simulink model "NUgus"  (R2018a)
settings: Solver=VariableStepAuto  StartTime=0.0  StopTime=inf  RelTol=1e-2
values from neighbouring files (symbols this model uses):
  CM740_acc_bias = 4 * 9.80743    (= 39.22972)    [CM740_init.m]
  CM740_acc_gain = 512 / CM740_acc_centre    [CM740_init.m]
  CM740_gyro_bias = 1600 / 360 * 2 * pi    (= 27.9252680319)    [CM740_init.m]
  CM740_gyro_gain = 512 / CM740_gyro_centre    [CM740_init.m]
  g = 9.8107    [init.m]
  head = [-0.05482228998067195, -0.00010888238321339966, 0.0011712900228573724, 0.41900000000000004]    [comtest.m]
  Kw = 0.9    [init.m]
  model = NUgusKinematics()    [KinematicsTest.m]    (also in Support_Region.m; init.m = NUgusKinematics)
  period = 1.0    (= 1)    [init.m]
  s = mean(abs(present_speed.data))    [RunServoTest.m]
  sample_time = 1/90    (= 0.0111111111111)    [init.m]
  step_height = 0.1    [init.m]
  torso = [0.0050079703254699804, 0.008880921777563762, 0.1021503146237477, 2.5390000000000006]    [comtest.m]
  z0 = 0.45    [init.m]
undefined symbols (not defined in the file or in its folder): sigbuilder_block, X, Y, Z
libraries: sm_lib x206, nesl_utility x82, Contact_Forces_Lib x10
(part 6 of 7)

== system NUgus/NUgus/right_upper_arm ==
  Inertia : sm_lib/Body Elements/Inertia  InertiaType=Custom  Mass=model.mass.arm_upper(4)  MassUnits=kg  CenterOfMass=[0, 0, 0]  CenterOfMassUnits=m  MomentsOfInertia=[model.inertia.upper_arm(1,1), model.inertia.upper_arm(2,2), model.inertia.upper_arm(3,3)]  MomentsOfInertiaUnits=kg*m^2  ProductsOfInertia=-[model.inertia.upper_arm(2,3), model.inertia.upper_arm(3,1), model.inertia.upper_arm(1,2)]  ProductsOfInertiaUnits=kg*m^2  GraphicType=Marker  MarkerShape=Inertia  MarkerSize=20  GraphicVisPropType=SimpleVisualProperties  GraphicDiffuseColor=[0.8 0.8 0.8]  GraphicSpecularColor=[0.5 0.5 0.5 1.0]  GraphicAmbientColor=[0.15 0.15 0.15 1.0]  GraphicEmissiveColor=[0.0 0.0 0.0 1.0]  GraphicShininess=75  GraphicOpacity=inertia_opacity
  InertiaOriginTransform : sm_lib/Frames and Transforms/Rigid Transform  TranslationMethod=Cartesian  TranslationStandardOffset=0  TranslationLengthUnit=m  TranslationStandardAxis=+Z  TranslationCartesianOffset=[0.006723 -0.090631 0.000549]  TranslationROffset=0  TranslationROffsetUnits=m  TranslationZOffset=0  TranslationZOffsetUnits=m  TranslationThetaOffset=0  TranslationThetaOffsetUnits=deg  RotationMethod=RotationSequence  RotationAngleUnits=deg  RotationStandardAxis=+Z  RotationAngle=0.0  RotationArbitraryAxis=[0 0 1]  FollAlignAxisA=+X  BaseAlignAxisA=+Y  FollAlignAxisB=+Y  BaseAlignAxisB=+Z  RotationSequenceAxes=BaseAxes  RotationSequence=XYZ  RotationSequenceAngles=[0, 0, 0]  RotationSequenceAnglesUnits=rad  RotationMatrix=[1 0 0; 0 1 0; 0 0 1]
  ReferenceFrame : sm_lib/Frames and Transforms/Reference Frame
  right_elbow_pitch_AxisTransform : sm_lib/Frames and Transforms/Rigid Transform  TranslationMethod=Cartesian  TranslationStandardOffset=0  TranslationLengthUnit=m  TranslationStandardAxis=+Z  TranslationCartesianOffset=[0, 0, 0]  TranslationROffset=0  TranslationROffsetUnits=m  TranslationZOffset=0  TranslationZOffsetUnits=m  TranslationThetaOffset=0  TranslationThetaOffsetUnits=deg  RotationMethod=ArbitraryAxis  RotationAngleUnits=rad  RotationStandardAxis=+Z  RotationAngle=1.570796326794897  RotationArbitraryAxis=[-0, 1, 0]  FollAlignAxisA=+X  BaseAlignAxisA=+Y  FollAlignAxisB=+Y  BaseAlignAxisB=+Z  RotationSequenceAxes=FollowerAxes  RotationSequence=XYX  RotationSequenceAngles=[0 0 0]  RotationSequenceAnglesUnits=deg  RotationMatrix=[1 0 0; 0 1 0; 0 0 1]
  right_elbow_pitch_OriginTransform : sm_lib/Frames and Transforms/Rigid Transform  TranslationMethod=Cartesian  TranslationStandardOffset=0  TranslationLengthUnit=m  TranslationStandardAxis=+Z  TranslationCartesianOffset=[0.01, -0.19, 0.04]  TranslationROffset=0  TranslationROffsetUnits=m  TranslationZOffset=0  TranslationZOffsetUnits=m  TranslationThetaOffset=0  TranslationThetaOffsetUnits=deg  RotationMethod=RotationSequence  RotationAngleUnits=deg  RotationStandardAxis=+Z  RotationAngle=0.0  RotationArbitraryAxis=[0 0 1]  FollAlignAxisA=+X  BaseAlignAxisA=+Y  FollAlignAxisB=+Y  BaseAlignAxisB=+Z  RotationSequenceAxes=BaseAxes  RotationSequence=XYZ  RotationSequenceAngles=[0, 0, 0]  RotationSequenceAnglesUnits=rad  RotationMatrix=[1 0 0; 0 1 0; 0 0 1]
  right_shoulder_roll_AxisInvTransform : sm_lib/Frames and Transforms/Rigid Transform  TranslationMethod=Cartesian  TranslationStandardOffset=0  TranslationLengthUnit=m  TranslationStandardAxis=+Z  TranslationCartesianOffset=[0, 0, 0]  TranslationROffset=0  TranslationROffsetUnits=m  TranslationZOffset=0  TranslationZOffsetUnits=m  TranslationThetaOffset=0  TranslationThetaOffsetUnits=deg  RotationMethod=ArbitraryAxis  RotationAngleUnits=rad  RotationStandardAxis=+Z  RotationAngle=0  RotationArbitraryAxis=[1, 0, 0]  FollAlignAxisA=+X  BaseAlignAxisA=+Y  FollAlignAxisB=+Y  BaseAlignAxisB=+Z  RotationSequenceAxes=FollowerAxes  RotationSequence=XYX  RotationSequenceAngles=[0 0 0]  RotationSequenceAnglesUnits=deg  RotationMatrix=[1 0 0; 0 1 0; 0 0 1]
  right_upper_arm_visual : sm_lib/Body Elements/Solid  InertiaType=Custom  Mass=0  MassUnits=kg  CenterOfMass=[0, 0, 0]  CenterOfMassUnits=m  MomentsOfInertia=[0, 0, 0]  MomentsOfInertiaUnits=kg*m^2  ProductsOfInertia=[0, 0, 0]  ProductsOfInertiaUnits=kg*m^2  DensityBased=on  Density=1000  DensityUnits=kg/m^3  DoExposeReferenceFrame=on  SerializedFrames=<Frames/>  GraphicType=FromGeometry  MarkerShape=Sphere  MarkerSize=10  GraphicVisPropType=SimpleVisualProperties  GraphicDiffuseColor=[0.5, 0.5, 0.5]  GraphicSpecularColor=[0.5 0.5 0.5 1.0]  GraphicAmbientColor=[0.15 0.15 0.15 1.0]  GraphicEmissiveColor=[0.0 0.0 0.0 1.0]  GraphicShininess=75  GraphicOpacity=1  GeometryShape=FromFile  RectangleSize=[1 1]  RectangleSizeUnits=m  BrickDimensions=[1 1 1]  BrickDimensionUnits=m  CylinderRadius=1  CylinderRadiusUnits=m  CylinderLength=1  CylinderLengthUnits=m  SphereRadius=1  SphereRadiusUnits=m  EllipsoidRadii=[1 1 1]  EllipsoidRadiiUnits=m  ExtrusionCrossSection=[1 1; -1 1; -1 -1; 1 -1]  ExtrusionCrossSectionUnits=m  ExtrusionLength=1  ExtrusionLengthUnits=m  PolygonNumSides=3  PolygonOuterRadius=1  PolygonOuterRadiusUnits=m  ExtGeomFileType=STL  ExtGeomFileName=mesh/right_upper_arm.stl  ExtGeomFileUnits=m  RevolutionCrossSection=[1 1; 1 -1; 2 -1; 2 1]  RevolutionCrossSectionUnits=m  RevolutionExtent=Full  RevolutionAngle=180  RevolutionAngleUnits=deg
  right_upper_arm_visualOriginTransform : sm_lib/Frames and Transforms/Rigid Transform  TranslationMethod=Cartesian  TranslationStandardOffset=0  TranslationLengthUnit=m  TranslationStandardAxis=+Z  TranslationCartesianOffset=[0, 0, 0]  TranslationROffset=0  TranslationROffsetUnits=m  TranslationZOffset=0  TranslationZOffsetUnits=m  TranslationThetaOffset=0  TranslationThetaOffsetUnits=deg  RotationMethod=RotationSequence  RotationAngleUnits=deg  RotationStandardAxis=+Z  RotationAngle=0.0  RotationArbitraryAxis=[0 0 1]  FollAlignAxisA=+X  BaseAlignAxisA=+Y  FollAlignAxisB=+Y  BaseAlignAxisB=+Z  RotationSequenceAxes=BaseAxes  RotationSequence=XYZ  RotationSequenceAngles=[0, 0, 0]  RotationSequenceAnglesUnits=rad  RotationMatrix=[1 0 0; 0 1 0; 0 0 1]
  F : PMIOPort  Side=Left
  F1 : PMIOPort  Port=2  Side=Right
  connections:
  Inertia/RConn1 -- InertiaOriginTransform/RConn1
  ReferenceFrame/RConn1 -- InertiaOriginTransform/LConn1 -- right_elbow_pitch_OriginTransform/LConn1 -- right_shoulder_roll_AxisInvTransform/LConn1 -- right_upper_arm_visualOriginTransform/LConn1
  right_elbow_pitch_AxisTransform/RConn1 -- F1/RConn1
  right_elbow_pitch_AxisTransform/LConn1 -- right_elbow_pitch_OriginTransform/RConn1
  right_shoulder_roll_AxisInvTransform/RConn1 -- F/RConn1
  right_upper_arm_visual/RConn1 -- right_upper_arm_visualOriginTransform/RConn1

== system NUgus/NUgus/right_upper_leg ==
  Inertia : sm_lib/Body Elements/Inertia  InertiaType=Custom  Mass=model.mass.leg_upper(4)  MassUnits=kg  CenterOfMass=[0, 0, 0]  CenterOfMassUnits=m  MomentsOfInertia=[model.inertia.upper_leg(1,1), model.inertia.upper_leg(2,2), model.inertia.upper_leg(3,3)]  MomentsOfInertiaUnits=kg*m^2  ProductsOfInertia=-[model.inertia.upper_leg(2,3), model.inertia.upper_leg(3,1), model.inertia.upper_leg(1,2)]  ProductsOfInertiaUnits=kg*m^2  GraphicType=Marker  MarkerShape=Inertia  MarkerSize=20  GraphicVisPropType=SimpleVisualProperties  GraphicDiffuseColor=[0.8 0.8 0.8]  GraphicSpecularColor=[0.5 0.5 0.5 1.0]  GraphicAmbientColor=[0.15 0.15 0.15 1.0]  GraphicEmissiveColor=[0.0 0.0 0.0 1.0]  GraphicShininess=75  GraphicOpacity=inertia_opacity
  InertiaOriginTransform : sm_lib/Frames and Transforms/Rigid Transform  TranslationMethod=Cartesian  TranslationStandardOffset=0  TranslationLengthUnit=m  TranslationStandardAxis=+Z  TranslationCartesianOffset=[0.000592 -0.005444 -0.102193]  TranslationROffset=0  TranslationROffsetUnits=m  TranslationZOffset=0  TranslationZOffsetUnits=m  TranslationThetaOffset=0  TranslationThetaOffsetUnits=deg  RotationMethod=RotationSequence  RotationAngleUnits=deg  RotationStandardAxis=+Z  RotationAngle=0.0  RotationArbitraryAxis=[0 0 1]  FollAlignAxisA=+X  BaseAlignAxisA=+Y  FollAlignAxisB=+Y  BaseAlignAxisB=+Z  RotationSequenceAxes=BaseAxes  RotationSequence=XYZ  RotationSequenceAngles=[0, 0, 0]  RotationSequenceAnglesUnits=rad  RotationMatrix=[1 0 0; 0 1 0; 0 0 1]
  ReferenceFrame : sm_lib/Frames and Transforms/Reference Frame
  right_hip_pitch_AxisInvTransform : sm_lib/Frames and Transforms/Rigid Transform  TranslationMethod=Cartesian  TranslationStandardOffset=0  TranslationLengthUnit=m  TranslationStandardAxis=+Z  TranslationCartesianOffset=[0, 0, 0]  TranslationROffset=0  TranslationROffsetUnits=m  TranslationZOffset=0  TranslationZOffsetUnits=m  TranslationThetaOffset=0  TranslationThetaOffsetUnits=deg  RotationMethod=ArbitraryAxis  RotationAngleUnits=rad  RotationStandardAxis=+Z  RotationAngle=1.570796326794897  RotationArbitraryAxis=[-0, 1, 0]  FollAlignAxisA=+X  BaseAlignAxisA=+Y  FollAlignAxisB=+Y  BaseAlignAxisB=+Z  RotationSequenceAxes=FollowerAxes  RotationSequence=XYX  RotationSequenceAngles=[0 0 0]  RotationSequenceAnglesUnits=deg  RotationMatrix=[1 0 0; 0 1 0; 0 0 1]
  right_knee_pitch_AxisTransform : sm_lib/Frames and Transforms/Rigid Transform  TranslationMethod=Cartesian  TranslationStandardOffset=0  TranslationLengthUnit=m  TranslationStandardAxis=+Z  TranslationCartesianOffset=[0, 0, 0]  TranslationROffset=0  TranslationROffsetUnits=m  TranslationZOffset=0  TranslationZOffsetUnits=m  TranslationThetaOffset=0  TranslationThetaOffsetUnits=deg  RotationMethod=ArbitraryAxis  RotationAngleUnits=rad  RotationStandardAxis=+Z  RotationAngle=1.570796326794897  RotationArbitraryAxis=[-0, 1, 0]  FollAlignAxisA=+X  BaseAlignAxisA=+Y  FollAlignAxisB=+Y  BaseAlignAxisB=+Z  RotationSequenceAxes=FollowerAxes  RotationSequence=XYX  RotationSequenceAngles=[0 0 0]  RotationSequenceAnglesUnits=deg  RotationMatrix=[1 0 0; 0 1 0; 0 0 1]
  right_knee_pitch_OriginTransform : sm_lib/Frames and Transforms/Rigid Transform  TranslationMethod=Cartesian  TranslationStandardOffset=0  TranslationLengthUnit=m  TranslationStandardAxis=+Z  TranslationCartesianOffset=[0, 0, -0.18976]  TranslationROffset=0  TranslationROffsetUnits=m  TranslationZOffset=0  TranslationZOffsetUnits=m  TranslationThetaOffset=0  TranslationThetaOffsetUnits=deg  RotationMethod=RotationSequence  RotationAngleUnits=deg  RotationStandardAxis=+Z  RotationAngle=0.0  RotationArbitraryAxis=[0 0 1]  FollAlignAxisA=+X  BaseAlignAxisA=+Y  FollAlignAxisB=+Y  BaseAlignAxisB=+Z  RotationSequenceAxes=BaseAxes  RotationSequence=XYZ  RotationSequenceAngles=[0.05, 0, 0]  RotationSequenceAnglesUnits=rad  RotationMatrix=[1 0 0; 0 1 0; 0 0 1]
  right_upper_leg_visual : sm_lib/Body Elements/Solid  InertiaType=Custom  Mass=0  MassUnits=kg  CenterOfMass=[0, 0, 0]  CenterOfMassUnits=m  MomentsOfInertia=[0, 0, 0]  MomentsOfInertiaUnits=kg*m^2  ProductsOfInertia=[0, 0, 0]  ProductsOfInertiaUnits=kg*m^2  DensityBased=on  Density=1000  DensityUnits=kg/m^3  DoExposeReferenceFrame=on  SerializedFrames=<Frames/>  GraphicType=FromGeometry  MarkerShape=Sphere  MarkerSize=10  GraphicVisPropType=SimpleVisualProperties  GraphicDiffuseColor=[0.5, 0.5, 0.5]  GraphicSpecularColor=[0.5 0.5 0.5 1.0]  GraphicAmbientColor=[0.15 0.15 0.15 1.0]  GraphicEmissiveColor=[0.0 0.0 0.0 1.0]  GraphicShininess=75  GraphicOpacity=1  GeometryShape=FromFile  RectangleSize=[1 1]  RectangleSizeUnits=m  BrickDimensions=[1 1 1]  BrickDimensionUnits=m  CylinderRadius=1  CylinderRadiusUnits=m  CylinderLength=1  CylinderLengthUnits=m  SphereRadius=1  SphereRadiusUnits=m  EllipsoidRadii=[1 1 1]  EllipsoidRadiiUnits=m  ExtrusionCrossSection=[1 1; -1 1; -1 -1; 1 -1]  ExtrusionCrossSectionUnits=m  ExtrusionLength=1  ExtrusionLengthUnits=m  PolygonNumSides=3  PolygonOuterRadius=1  PolygonOuterRadiusUnits=m  ExtGeomFileType=STL  ExtGeomFileName=mesh/right_upper_leg.stl  ExtGeomFileUnits=m  RevolutionCrossSection=[1 1; 1 -1; 2 -1; 2 1]  RevolutionCrossSectionUnits=m  RevolutionExtent=Full  RevolutionAngle=180  RevolutionAngleUnits=deg
  right_upper_leg_visualOriginTransform : sm_lib/Frames and Transforms/Rigid Transform  TranslationMethod=Cartesian  TranslationStandardOffset=0  TranslationLengthUnit=m  TranslationStandardAxis=+Z  TranslationCartesianOffset=[0, 0, 0]  TranslationROffset=0  TranslationROffsetUnits=m  TranslationZOffset=0  TranslationZOffsetUnits=m  TranslationThetaOffset=0  TranslationThetaOffsetUnits=deg  RotationMethod=RotationSequence  RotationAngleUnits=deg  RotationStandardAxis=+Z  RotationAngle=0.0  RotationArbitraryAxis=[0 0 1]  FollAlignAxisA=+X  BaseAlignAxisA=+Y  FollAlignAxisB=+Y  BaseAlignAxisB=+Z  RotationSequenceAxes=BaseAxes  RotationSequence=XYZ  RotationSequenceAngles=[0, 0, 0]  RotationSequenceAnglesUnits=rad  RotationMatrix=[1 0 0; 0 1 0; 0 0 1]
  F : PMIOPort  Side=Left
  F1 : PMIOPort  Port=2  Side=Right
  connections:
  Inertia/RConn1 -- InertiaOriginTransform/RConn1
  ReferenceFrame/RConn1 -- InertiaOriginTransform/LConn1 -- right_hip_pitch_AxisInvTransform/LConn1 -- right_knee_pitch_OriginTransform/LConn1 -- right_upper_leg_visualOriginTransform/LConn1
  right_hip_pitch_AxisInvTransform/RConn1 -- F/RConn1
  right_knee_pitch_AxisTransform/RConn1 -- F1/RConn1
  right_knee_pitch_AxisTransform/LConn1 -- right_knee_pitch_OriginTransform/RConn1
  right_upper_leg_visual/RConn1 -- right_upper_leg_visualOriginTransform/RConn1

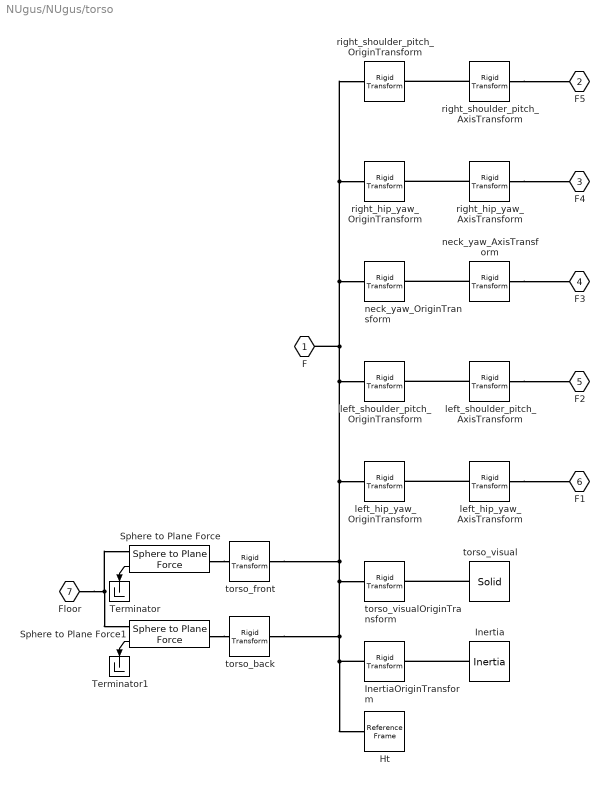
== system NUgus/NUgus/torso ==
  Ht : sm_lib/Frames and Transforms/Reference Frame
  Inertia : sm_lib/Body Elements/Inertia  InertiaType=Custom  Mass=model.mass.torso(4)  MassUnits=kg  CenterOfMass=[0, 0, 0]  CenterOfMassUnits=m  MomentsOfInertia=[model.inertia.torso(1,1), model.inertia.torso(2,2), model.inertia.torso(3,3)]  MomentsOfInertiaUnits=kg*m^2  ProductsOfInertia=-[model.inertia.torso(2,3), model.inertia.torso(3,1), model.inertia.torso(1,2)]  ProductsOfInertiaUnits=kg*m^2  GraphicType=Marker  MarkerShape=Inertia  MarkerSize=20  GraphicVisPropType=SimpleVisualProperties  GraphicDiffuseColor=[0.8 0.8 0.8]  GraphicSpecularColor=[0.5 0.5 0.5 1.0]  GraphicAmbientColor=[0.15 0.15 0.15 1.0]  GraphicEmissiveColor=[0.0 0.0 0.0 1.0]  GraphicShininess=75  GraphicOpacity=inertia_opacity
  InertiaOriginTransform : sm_lib/Frames and Transforms/Rigid Transform  TranslationMethod=Cartesian  TranslationStandardOffset=0  TranslationLengthUnit=m  TranslationStandardAxis=+Z  TranslationCartesianOffset=[-0.000000 0.000339 0.112557]  TranslationROffset=0  TranslationROffsetUnits=m  TranslationZOffset=0  TranslationZOffsetUnits=m  TranslationThetaOffset=0  TranslationThetaOffsetUnits=deg  RotationMethod=RotationSequence  RotationAngleUnits=deg  RotationStandardAxis=+Z  RotationAngle=0.0  RotationArbitraryAxis=[0 0 1]  FollAlignAxisA=+X  BaseAlignAxisA=+Y  FollAlignAxisB=+Y  BaseAlignAxisB=+Z  RotationSequenceAxes=BaseAxes  RotationSequence=XYZ  RotationSequenceAngles=[0, 0, 0]  RotationSequenceAnglesUnits=rad  RotationMatrix=[1 0 0; 0 1 0; 0 0 1]
  Sphere to Plane Force : Contact_Forces_Lib/3D/Sphere to Plane Force  sphere_rad=floor.stud_radius  plane_lenx=floor.length  plane_leny=floor.width  plane_depth=floor.depth/2  force_law=Linear  k_contact=floor.contact_stiffness  b_contact=floor.contact_damping  pen_full_damp_F=1e-4  pen_exponent=1  custom_param_1=1  custom_param_2=1  friction_law=Stick-Slip Continuous  mu_kinetic=floor.kinetic_friction  mu_static=floor.static_friction  v_thr=floor.vel_gain  vis_on=off  vis_opc_en=0  vis_len_plaBz=0.005  vis_clr=[0.9 0.2 0.2]  vis_opc=0.7
  Sphere to Plane Force1 : Contact_Forces_Lib/3D/Sphere to Plane Force  sphere_rad=floor.stud_radius  plane_lenx=floor.length  plane_leny=floor.width  plane_depth=floor.depth/2  force_law=Linear  k_contact=floor.contact_stiffness  b_contact=floor.contact_damping  pen_full_damp_F=1e-4  pen_exponent=1  custom_param_1=1  custom_param_2=1  friction_law=Stick-Slip Continuous  mu_kinetic=floor.kinetic_friction  mu_static=floor.static_friction  v_thr=floor.vel_gain  vis_on=off  vis_opc_en=0  vis_len_plaBz=0.005  vis_clr=[0.9 0.2 0.2]  vis_opc=0.7
  Terminator : Terminator
  Terminator1 : Terminator
  left_hip_yaw_AxisTransform : sm_lib/Frames and Transforms/Rigid Transform  TranslationMethod=Cartesian  TranslationStandardOffset=0  TranslationLengthUnit=m  TranslationStandardAxis=+Z  TranslationCartesianOffset=[0, 0, 0]  TranslationROffset=0  TranslationROffsetUnits=m  TranslationZOffset=0  TranslationZOffsetUnits=m  TranslationThetaOffset=0  TranslationThetaOffsetUnits=deg  RotationMethod=ArbitraryAxis  RotationAngleUnits=rad  RotationStandardAxis=+Z  RotationAngle=0  RotationArbitraryAxis=[1, 0, 0]  FollAlignAxisA=+X  BaseAlignAxisA=+Y  FollAlignAxisB=+Y  BaseAlignAxisB=+Z  RotationSequenceAxes=FollowerAxes  RotationSequence=XYX  RotationSequenceAngles=[0 0 0]  RotationSequenceAnglesUnits=deg  RotationMatrix=[1 0 0; 0 1 0; 0 0 1]
  left_hip_yaw_OriginTransform : sm_lib/Frames and Transforms/Rigid Transform  TranslationMethod=Cartesian  TranslationStandardOffset=0  TranslationLengthUnit=m  TranslationStandardAxis=+Z  TranslationCartesianOffset=[0, 0.055, 0]  TranslationROffset=0  TranslationROffsetUnits=m  TranslationZOffset=0  TranslationZOffsetUnits=m  TranslationThetaOffset=0  TranslationThetaOffsetUnits=deg  RotationMethod=RotationSequence  RotationAngleUnits=deg  RotationStandardAxis=+Z  RotationAngle=0.0  RotationArbitraryAxis=[0 0 1]  FollAlignAxisA=+X  BaseAlignAxisA=+Y  FollAlignAxisB=+Y  BaseAlignAxisB=+Z  RotationSequenceAxes=BaseAxes  RotationSequence=XYZ  RotationSequenceAngles=[0, 0, 1.57079]  RotationSequenceAnglesUnits=rad  RotationMatrix=[1 0 0; 0 1 0; 0 0 1]
  left_shoulder_pitch_AxisTransform : sm_lib/Frames and Transforms/Rigid Transform  TranslationMethod=Cartesian  TranslationStandardOffset=0  TranslationLengthUnit=m  TranslationStandardAxis=+Z  TranslationCartesianOffset=[0, 0, 0]  TranslationROffset=0  TranslationROffsetUnits=m  TranslationZOffset=0  TranslationZOffsetUnits=m  TranslationThetaOffset=0  TranslationThetaOffsetUnits=deg  RotationMethod=ArbitraryAxis  RotationAngleUnits=rad  RotationStandardAxis=+Z  RotationAngle=1.570796326794897  RotationArbitraryAxis=[-0, 1, 0]  FollAlignAxisA=+X  BaseAlignAxisA=+Y  FollAlignAxisB=+Y  BaseAlignAxisB=+Z  RotationSequenceAxes=FollowerAxes  RotationSequence=XYX  RotationSequenceAngles=[0 0 0]  RotationSequenceAnglesUnits=deg  RotationMatrix=[1 0 0; 0 1 0; 0 0 1]
  left_shoulder_pitch_OriginTransform : sm_lib/Frames and Transforms/Rigid Transform  TranslationMethod=Cartesian  TranslationStandardOffset=0  TranslationLengthUnit=m  TranslationStandardAxis=+Z  TranslationCartesianOffset=[0.005, 0.115, 0.18]  TranslationROffset=0  TranslationROffsetUnits=m  TranslationZOffset=0  TranslationZOffsetUnits=m  TranslationThetaOffset=0  TranslationThetaOffsetUnits=deg  RotationMethod=RotationSequence  RotationAngleUnits=deg  RotationStandardAxis=+Z  RotationAngle=0.0  RotationArbitraryAxis=[0 0 1]  FollAlignAxisA=+X  BaseAlignAxisA=+Y  FollAlignAxisB=+Y  BaseAlignAxisB=+Z  RotationSequenceAxes=BaseAxes  RotationSequence=XYZ  RotationSequenceAngles=[-1.57079, 0, 1.57079]  RotationSequenceAnglesUnits=rad  RotationMatrix=[1 0 0; 0 1 0; 0 0 1]
  neck_yaw_AxisTransform : sm_lib/Frames and Transforms/Rigid Transform  TranslationMethod=Cartesian  TranslationStandardOffset=0  TranslationLengthUnit=m  TranslationStandardAxis=+Z  TranslationCartesianOffset=[0, 0, 0]  TranslationROffset=0  TranslationROffsetUnits=m  TranslationZOffset=0  TranslationZOffsetUnits=m  TranslationThetaOffset=0  TranslationThetaOffsetUnits=deg  RotationMethod=ArbitraryAxis  RotationAngleUnits=rad  RotationStandardAxis=+Z  RotationAngle=0  RotationArbitraryAxis=[1, 0, 0]  FollAlignAxisA=+X  BaseAlignAxisA=+Y  FollAlignAxisB=+Y  BaseAlignAxisB=+Z  RotationSequenceAxes=FollowerAxes  RotationSequence=XYX  RotationSequenceAngles=[0 0 0]  RotationSequenceAnglesUnits=deg  RotationMatrix=[1 0 0; 0 1 0; 0 0 1]
  neck_yaw_OriginTransform : sm_lib/Frames and Transforms/Rigid Transform  TranslationMethod=Cartesian  TranslationStandardOffset=0  TranslationLengthUnit=m  TranslationStandardAxis=+Z  TranslationCartesianOffset=[0, 0, 0.26]  TranslationROffset=0  TranslationROffsetUnits=m  TranslationZOffset=0  TranslationZOffsetUnits=m  TranslationThetaOffset=0  TranslationThetaOffsetUnits=deg  RotationMethod=RotationSequence  RotationAngleUnits=deg  RotationStandardAxis=+Z  RotationAngle=0.0  RotationArbitraryAxis=[0 0 1]  FollAlignAxisA=+X  BaseAlignAxisA=+Y  FollAlignAxisB=+Y  BaseAlignAxisB=+Z  RotationSequenceAxes=BaseAxes  RotationSequence=XYZ  RotationSequenceAngles=[0, 0, 1.57079]  RotationSequenceAnglesUnits=rad  RotationMatrix=[1 0 0; 0 1 0; 0 0 1]
  right_hip_yaw_AxisTransform : sm_lib/Frames and Transforms/Rigid Transform  TranslationMethod=Cartesian  TranslationStandardOffset=0  TranslationLengthUnit=m  TranslationStandardAxis=+Z  TranslationCartesianOffset=[0, 0, 0]  TranslationROffset=0  TranslationROffsetUnits=m  TranslationZOffset=0  TranslationZOffsetUnits=m  TranslationThetaOffset=0  TranslationThetaOffsetUnits=deg  RotationMethod=ArbitraryAxis  RotationAngleUnits=rad  RotationStandardAxis=+Z  RotationAngle=0  RotationArbitraryAxis=[1, 0, 0]  FollAlignAxisA=+X  BaseAlignAxisA=+Y  FollAlignAxisB=+Y  BaseAlignAxisB=+Z  RotationSequenceAxes=FollowerAxes  RotationSequence=XYX  RotationSequenceAngles=[0 0 0]  RotationSequenceAnglesUnits=deg  RotationMatrix=[1 0 0; 0 1 0; 0 0 1]
  right_hip_yaw_OriginTransform : sm_lib/Frames and Transforms/Rigid Transform  TranslationMethod=Cartesian  TranslationStandardOffset=0  TranslationLengthUnit=m  TranslationStandardAxis=+Z  TranslationCartesianOffset=[0, -0.055, 0]  TranslationROffset=0  TranslationROffsetUnits=m  TranslationZOffset=0  TranslationZOffsetUnits=m  TranslationThetaOffset=0  TranslationThetaOffsetUnits=deg  RotationMethod=RotationSequence  RotationAngleUnits=deg  RotationStandardAxis=+Z  RotationAngle=0.0  RotationArbitraryAxis=[0 0 1]  FollAlignAxisA=+X  BaseAlignAxisA=+Y  FollAlignAxisB=+Y  BaseAlignAxisB=+Z  RotationSequenceAxes=BaseAxes  RotationSequence=XYZ  RotationSequenceAngles=[0, 0, 1.57079]  RotationSequenceAnglesUnits=rad  RotationMatrix=[1 0 0; 0 1 0; 0 0 1]
  right_shoulder_pitch_AxisTransform : sm_lib/Frames and Transforms/Rigid Transform  TranslationMethod=Cartesian  TranslationStandardOffset=0  TranslationLengthUnit=m  TranslationStandardAxis=+Z  TranslationCartesianOffset=[0, 0, 0]  TranslationROffset=0  TranslationROffsetUnits=m  TranslationZOffset=0  TranslationZOffsetUnits=m  TranslationThetaOffset=0  TranslationThetaOffsetUnits=deg  RotationMethod=ArbitraryAxis  RotationAngleUnits=rad  RotationStandardAxis=+Z  RotationAngle=1.570796326794897  RotationArbitraryAxis=[-0, 1, 0]  FollAlignAxisA=+X  BaseAlignAxisA=+Y  FollAlignAxisB=+Y  BaseAlignAxisB=+Z  RotationSequenceAxes=FollowerAxes  RotationSequence=XYX  RotationSequenceAngles=[0 0 0]  RotationSequenceAnglesUnits=deg  RotationMatrix=[1 0 0; 0 1 0; 0 0 1]
  right_shoulder_pitch_OriginTransform : sm_lib/Frames and Transforms/Rigid Transform  TranslationMethod=Cartesian  TranslationStandardOffset=0  TranslationLengthUnit=m  TranslationStandardAxis=+Z  TranslationCartesianOffset=[0.005, -0.115, 0.18]  TranslationROffset=0  TranslationROffsetUnits=m  TranslationZOffset=0  TranslationZOffsetUnits=m  TranslationThetaOffset=0  TranslationThetaOffsetUnits=deg  RotationMethod=RotationSequence  RotationAngleUnits=deg  RotationStandardAxis=+Z  RotationAngle=0.0  RotationArbitraryAxis=[0 0 1]  FollAlignAxisA=+X  BaseAlignAxisA=+Y  FollAlignAxisB=+Y  BaseAlignAxisB=+Z  RotationSequenceAxes=BaseAxes  RotationSequence=XYZ  RotationSequenceAngles=[-1.57079, 0, 1.57079]  RotationSequenceAnglesUnits=rad  RotationMatrix=[1 0 0; 0 1 0; 0 0 1]
  torso_back : sm_lib/Frames and Transforms/Rigid Transform  TranslationMethod=Cartesian  TranslationStandardOffset=0  TranslationLengthUnit=m  TranslationStandardAxis=+Z  TranslationCartesianOffset=[-0.069 0 0.15]  TranslationROffset=0  TranslationROffsetUnits=m  TranslationZOffset=0  TranslationZOffsetUnits=m  TranslationThetaOffset=0  TranslationThetaOffsetUnits=deg  RotationMethod=None  RotationAngleUnits=deg  RotationStandardAxis=+Z  RotationAngle=0.0  RotationArbitraryAxis=[0 0 1]  FollAlignAxisA=+X  BaseAlignAxisA=+Y  FollAlignAxisB=+Y  BaseAlignAxisB=+Z  RotationSequenceAxes=FollowerAxes  RotationSequence=XYX  RotationSequenceAngles=[0 0 0]  RotationSequenceAnglesUnits=deg  RotationMatrix=[1 0 0; 0 1 0; 0 0 1]
  torso_front : sm_lib/Frames and Transforms/Rigid Transform  TranslationMethod=Cartesian  TranslationStandardOffset=0  TranslationLengthUnit=m  TranslationStandardAxis=+Z  TranslationCartesianOffset=[0.067 0 0.15]  TranslationROffset=0  TranslationROffsetUnits=m  TranslationZOffset=0  TranslationZOffsetUnits=m  TranslationThetaOffset=0  TranslationThetaOffsetUnits=deg  RotationMethod=None  RotationAngleUnits=deg  RotationStandardAxis=+Z  RotationAngle=0.0  RotationArbitraryAxis=[0 0 1]  FollAlignAxisA=+X  BaseAlignAxisA=+Y  FollAlignAxisB=+Y  BaseAlignAxisB=+Z  RotationSequenceAxes=FollowerAxes  RotationSequence=XYX  RotationSequenceAngles=[0 0 0]  RotationSequenceAnglesUnits=deg  RotationMatrix=[1 0 0; 0 1 0; 0 0 1]
  torso_visual : sm_lib/Body Elements/Solid  InertiaType=Custom  Mass=0  MassUnits=kg  CenterOfMass=[0, 0, 0]  CenterOfMassUnits=m  MomentsOfInertia=[0, 0, 0]  MomentsOfInertiaUnits=kg*m^2  ProductsOfInertia=[0, 0, 0]  ProductsOfInertiaUnits=kg*m^2  DensityBased=on  Density=1000  DensityUnits=kg/m^3  DoExposeReferenceFrame=on  SerializedFrames=<Frames/>  GraphicType=FromGeometry  MarkerShape=Sphere  MarkerSize=10  GraphicVisPropType=SimpleVisualProperties  GraphicDiffuseColor=[0.5, 0.5, 0.5]  GraphicSpecularColor=[0.5 0.5 0.5 1.0]  GraphicAmbientColor=[0.15 0.15 0.15 1.0]  GraphicEmissiveColor=[0.0 0.0 0.0 1.0]  GraphicShininess=75  GraphicOpacity=1  GeometryShape=FromFile  RectangleSize=[1 1]  RectangleSizeUnits=m  BrickDimensions=[1 1 1]  BrickDimensionUnits=m  CylinderRadius=1  CylinderRadiusUnits=m  CylinderLength=1  CylinderLengthUnits=m  SphereRadius=1  SphereRadiusUnits=m  EllipsoidRadii=[1 1 1]  EllipsoidRadiiUnits=m  ExtrusionCrossSection=[1 1; -1 1; -1 -1; 1 -1]  ExtrusionCrossSectionUnits=m  ExtrusionLength=1  ExtrusionLengthUnits=m  PolygonNumSides=3  PolygonOuterRadius=1  PolygonOuterRadiusUnits=m  ExtGeomFileType=STL  ExtGeomFileName=mesh/torso.stl  ExtGeomFileUnits=m  RevolutionCrossSection=[1 1; 1 -1; 2 -1; 2 1]  RevolutionCrossSectionUnits=m  RevolutionExtent=Full  RevolutionAngle=180  RevolutionAngleUnits=deg
  torso_visualOriginTransform : sm_lib/Frames and Transforms/Rigid Transform  TranslationMethod=Cartesian  TranslationStandardOffset=0  TranslationLengthUnit=m  TranslationStandardAxis=+Z  TranslationCartesianOffset=[0, 0, 0]  TranslationROffset=0  TranslationROffsetUnits=m  TranslationZOffset=0  TranslationZOffsetUnits=m  TranslationThetaOffset=0  TranslationThetaOffsetUnits=deg  RotationMethod=RotationSequence  RotationAngleUnits=deg  RotationStandardAxis=+Z  RotationAngle=0.0  RotationArbitraryAxis=[0 0 1]  FollAlignAxisA=+X  BaseAlignAxisA=+Y  FollAlignAxisB=+Y  BaseAlignAxisB=+Z  RotationSequenceAxes=BaseAxes  RotationSequence=XYZ  RotationSequenceAngles=[0, 0, 1.57079]  RotationSequenceAnglesUnits=rad  RotationMatrix=[1 0 0; 0 1 0; 0 0 1]
  F : PMIOPort  Side=Left
  F5 : PMIOPort  Port=2  Side=Right
  F4 : PMIOPort  Port=3  Side=Right
  F3 : PMIOPort  Port=4  Side=Right
  F2 : PMIOPort  Port=5  Side=Right
  F1 : PMIOPort  Port=6  Side=Right
  Floor : PMIOPort  Port=7  Side=Left
  wires:
  Sphere to Plane Force/1 -> Terminator/1
  Sphere to Plane Force1/1 -> Terminator1/1
  connections:
  Inertia/RConn1 -- InertiaOriginTransform/RConn1
  InertiaOriginTransform/LConn1 -- Ht/RConn1 -- torso_back/LConn1 -- torso_front/LConn1 -- F/RConn1 -- right_hip_yaw_OriginTransform/LConn1 -- right_shoulder_pitch_OriginTransform/LConn1 -- neck_yaw_OriginTransform/LConn1 -- left_shoulder_pitch_OriginTransform/LConn1 -- left_hip_yaw_OriginTransform/LConn1 -- torso_visualOriginTransform/LConn1
  left_hip_yaw_AxisTransform/RConn1 -- F1/RConn1
  left_hip_yaw_AxisTransform/LConn1 -- left_hip_yaw_OriginTransform/RConn1
  left_shoulder_pitch_AxisTransform/RConn1 -- F2/RConn1
  left_shoulder_pitch_AxisTransform/LConn1 -- left_shoulder_pitch_OriginTransform/RConn1
  neck_yaw_AxisTransform/RConn1 -- F3/RConn1
  neck_yaw_AxisTransform/LConn1 -- neck_yaw_OriginTransform/RConn1
  right_hip_yaw_AxisTransform/RConn1 -- F4/RConn1
  right_hip_yaw_AxisTransform/LConn1 -- right_hip_yaw_OriginTransform/RConn1
  right_shoulder_pitch_AxisTransform/RConn1 -- F5/RConn1
  right_shoulder_pitch_AxisTransform/LConn1 -- right_shoulder_pitch_OriginTransform/RConn1
  torso_visual/RConn1 -- torso_visualOriginTransform/RConn1
  Sphere to Plane Force/LConn1 -- torso_front/RConn1
  Sphere to Plane Force1/LConn1 -- torso_back/RConn1
  Floor/RConn1 -- Sphere to Plane Force1/RConn1 -- Sphere to Plane Force/RConn1

== system NUgus/Control/Capture Step/Subsystem3 ==
  v3 : Inport
  Constant4 : Constant
  Demux5 : Demux  Outputs=3
  Mux2 : Mux
  v4 : Outport
  wires:
  Mux2/1 -> v4/1
  v3/1 -> Demux5/1
  Demux5/2 -> Mux2/2
  Demux5/3 -> Mux2/3
  Demux5/1 -> Mux2/1
  Constant4/1 -> Mux2/4

== system NUgus/Control/Capture Step/Subsystem4 ==
  v4 : Inport
  Demux5 : Demux
  Mux2 : Mux  Inputs=3
  Terminator : Terminator
  v3 : Outport
  wires:
  Mux2/1 -> v3/1
  v4/1 -> Demux5/1
  Demux5/2 -> Mux2/2
  Demux5/3 -> Mux2/3
  Demux5/1 -> Mux2/1
  Demux5/4 -> Terminator/1

== system NUgus/Control/ZMP/to real ==
  discrete : Inport
  Add : Sum  Inputs=+-
  Constant : Constant  Value=512
  Gain : Gain  Gain=(4 * 9.80657) / 512
  continuous : Outport
  wires:
  discrete/1 -> Add/1
  Add/1 -> Gain/1
  Gain/1 -> continuous/1
  Constant/1 -> Add/2

== system NUgus/Control/world to torso/Subsystem3 ==
  v3 : Inport
  Constant4 : Constant
  Demux5 : Demux  Outputs=3
  Mux2 : Mux
  v4 : Outport
  wires:
  Mux2/1 -> v4/1
  v3/1 -> Demux5/1
  Demux5/2 -> Mux2/2
  Demux5/3 -> Mux2/3
  Demux5/1 -> Mux2/1
  Constant4/1 -> Mux2/4

== system NUgus/Control/world to torso/Subsystem4 ==
  v4 : Inport
  Demux5 : Demux
  Mux2 : Mux  Inputs=3
  Terminator : Terminator
  v3 : Outport
  wires:
  Mux2/1 -> v3/1
  v4/1 -> Demux5/1
  Demux5/2 -> Mux2/2
  Demux5/3 -> Mux2/3
  Demux5/1 -> Mux2/1
  Demux5/4 -> Terminator/1

== system NUgus/Control/world to torso1/Subsystem3 ==
  v3 : Inport
  Constant4 : Constant
  Demux5 : Demux  Outputs=3
  Mux2 : Mux
  v4 : Outport
  wires:
  Mux2/1 -> v4/1
  v3/1 -> Demux5/1
  Demux5/2 -> Mux2/2
  Demux5/3 -> Mux2/3
  Demux5/1 -> Mux2/1
  Constant4/1 -> Mux2/4

== system NUgus/Control/world to torso1/Subsystem4 ==
  v4 : Inport
  Demux5 : Demux
  Mux2 : Mux  Inputs=3
  Terminator : Terminator
  v3 : Outport
  wires:
  Mux2/1 -> v3/1
  v4/1 -> Demux5/1
  Demux5/2 -> Mux2/2
  Demux5/3 -> Mux2/3
  Demux5/1 -> Mux2/1
  Demux5/4 -> Terminator/1

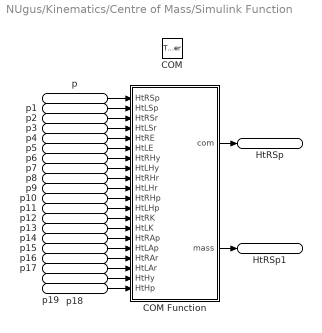
== system NUgus/Kinematics/Centre of Mass/Simulink Function ==
  COM : TriggerPort  TriggerType=function-call  IsSimulinkFunction=on  FunctionName=COM  FunctionVisibility=scoped  VariantControl=(inherit)
  COM Function : MATLAB Function  TreatAsAtomicUnit=on
  p : ArgIn  DisableCoverage=on  PortDimensions=[4 4]  ArgumentName=HtRSp
  p1 : ArgIn  DisableCoverage=on  Port=2  PortDimensions=[4 4]  ArgumentName=HtLSp
  p2 : ArgIn  DisableCoverage=on  Port=3  PortDimensions=[4 4]  ArgumentName=HtRSr
  p3 : ArgIn  DisableCoverage=on  Port=4  PortDimensions=[4 4]  ArgumentName=HtLSr
  p4 : ArgIn  DisableCoverage=on  Port=5  PortDimensions=[4 4]  ArgumentName=HtRE
  p5 : ArgIn  DisableCoverage=on  Port=6  PortDimensions=[4 4]  ArgumentName=HtLE
  p6 : ArgIn  DisableCoverage=on  Port=7  PortDimensions=[4 4]  ArgumentName=HtRHy
  p7 : ArgIn  DisableCoverage=on  Port=8  PortDimensions=[4 4]  ArgumentName=HtLHy
  p8 : ArgIn  DisableCoverage=on  Port=9  PortDimensions=[4 4]  ArgumentName=HtRHr
  p9 : ArgIn  DisableCoverage=on  Port=10  PortDimensions=[4 4]  ArgumentName=HtLHr
  p10 : ArgIn  DisableCoverage=on  Port=11  PortDimensions=[4 4]  ArgumentName=HtRHp
  p11 : ArgIn  DisableCoverage=on  Port=12  PortDimensions=[4 4]  ArgumentName=HtLHp
  p12 : ArgIn  DisableCoverage=on  Port=13  PortDimensions=[4 4]  ArgumentName=HtRK
  p13 : ArgIn  DisableCoverage=on  Port=14  PortDimensions=[4 4]  ArgumentName=HtLK
  p14 : ArgIn  DisableCoverage=on  Port=15  PortDimensions=[4 4]  ArgumentName=HtRAp
  p15 : ArgIn  DisableCoverage=on  Port=16  PortDimensions=[4 4]  ArgumentName=HtLAp
  p16 : ArgIn  DisableCoverage=on  Port=17  PortDimensions=[4 4]  ArgumentName=HtRAr
  p17 : ArgIn  DisableCoverage=on  Port=18  PortDimensions=[4 4]  ArgumentName=HtLAr
  p18 : ArgIn  DisableCoverage=on  Port=19  PortDimensions=[4 4]  ArgumentName=HtHy
  p19 : ArgIn  DisableCoverage=on  Port=20  PortDimensions=[4 4]  ArgumentName=HtHp
  HtRSp : ArgOut  DisableCoverage=on  PortDimensions=[1 3]  ArgumentName=com
  HtRSp1 : ArgOut  DisableCoverage=on  Port=2  ArgumentName=mass
  wires:
  p/1 -> COM Function/1(HtRSp)
  p1/1 -> COM Function/2(HtLSp)
  p2/1 -> COM Function/3(HtRSr)
  p3/1 -> COM Function/4(HtLSr)
  p4/1 -> COM Function/5(HtRE)
  p5/1 -> COM Function/6(HtLE)
  p6/1 -> COM Function/7(HtRHy)
  p7/1 -> COM Function/8(HtLHy)
  p8/1 -> COM Function/9(HtRHr)
  p9/1 -> COM Function/10(HtLHr)
  p10/1 -> COM Function/11(HtRHp)
  p11/1 -> COM Function/12(HtLHp)
  p12/1 -> COM Function/13(HtRK)
  p13/1 -> COM Function/14(HtLK)
  p14/1 -> COM Function/15(HtRAp)
  p15/1 -> COM Function/16(HtLAp)
  p16/1 -> COM Function/17(HtRAr)
  p17/1 -> COM Function/18(HtLAr)
  p18/1 -> COM Function/19(HtHy)
  p19/1 -> COM Function/20(HtHp)
  COM Function/1(com) -> HtRSp/1
  COM Function/2(mass) -> HtRSp1/1

== system NUgus/Kinematics/Forward Kinematics/Simulink Function ==
  FK : TriggerPort  TriggerType=function-call  IsSimulinkFunction=on  FunctionName=FK  FunctionVisibility=scoped  VariantControl=(inherit)
  FK Function : MATLAB Function  TreatAsAtomicUnit=on
  p : ArgIn  DisableCoverage=on  PortDimensions=[1 20]  ArgumentName=p
  HtRSp : ArgOut  DisableCoverage=on  PortDimensions=[4 4]  ArgumentName=HtRSp
  HtLSp : ArgOut  DisableCoverage=on  Port=2  PortDimensions=[4 4]  ArgumentName=HtLSp
  HtRSr : ArgOut  DisableCoverage=on  Port=3  PortDimensions=[4 4]  ArgumentName=HtRSr
  HtLSr : ArgOut  DisableCoverage=on  Port=4  PortDimensions=[4 4]  ArgumentName=HtLSr
  HtRE : ArgOut  DisableCoverage=on  Port=5  PortDimensions=[4 4]  ArgumentName=HtRE
  HtLE : ArgOut  DisableCoverage=on  Port=6  PortDimensions=[4 4]  ArgumentName=HtLE
  HtRHy : ArgOut  DisableCoverage=on  Port=7  PortDimensions=[4 4]  ArgumentName=HtRHy
  HtLHy : ArgOut  DisableCoverage=on  Port=8  PortDimensions=[4 4]  ArgumentName=HtLHy
  HtRHr : ArgOut  DisableCoverage=on  Port=9  PortDimensions=[4 4]  ArgumentName=HtRHr
  HtLHr : ArgOut  DisableCoverage=on  Port=10  PortDimensions=[4 4]  ArgumentName=HtLHr
  HtRHp : ArgOut  DisableCoverage=on  Port=11  PortDimensions=[4 4]  ArgumentName=HtRHp
  HtLHp : ArgOut  DisableCoverage=on  Port=12  PortDimensions=[4 4]  ArgumentName=HtLHp
  HtRK : ArgOut  DisableCoverage=on  Port=13  PortDimensions=[4 4]  ArgumentName=HtRK
  HtLK : ArgOut  DisableCoverage=on  Port=14  PortDimensions=[4 4]  ArgumentName=HtLK
  HtRAp : ArgOut  DisableCoverage=on  Port=15  PortDimensions=[4 4]  ArgumentName=HtRAp
  HtLAp : ArgOut  DisableCoverage=on  Port=16  PortDimensions=[4 4]  ArgumentName=HtLAp
  HtRAr : ArgOut  DisableCoverage=on  Port=17  PortDimensions=[4 4]  ArgumentName=HtRAr
  HtLAr : ArgOut  DisableCoverage=on  Port=18  PortDimensions=[4 4]  ArgumentName=HtLAr
  HtHy : ArgOut  DisableCoverage=on  Port=19  PortDimensions=[4 4]  ArgumentName=HtHy
  HtHp : ArgOut  DisableCoverage=on  Port=20  PortDimensions=[4 4]  ArgumentName=HtHp
  wires:
  p/1 -> FK Function/1(p)
  FK Function/15(HtRAp) -> HtRAp/1
  FK Function/10(HtLHr) -> HtLHr/1
  FK Function/9(HtRHr) -> HtRHr/1
  FK Function/8(HtLHy) -> HtLHy/1
  FK Function/7(HtRHy) -> HtRHy/1
  FK Function/2(HtLSp) -> HtLSp/1
  FK Function/14(HtLK) -> HtLK/1
  FK Function/3(HtRSr) -> HtRSr/1
  FK Function/6(HtLE) -> HtLE/1
  FK Function/5(HtRE) -> HtRE/1
  FK Function/1(HtRSp) -> HtRSp/1
  FK Function/16(HtLAp) -> HtLAp/1
  FK Function/17(HtRAr) -> HtRAr/1
  FK Function/19(HtHy) -> HtHy/1
  FK Function/4(HtLSr) -> HtLSr/1
  FK Function/20(HtHp) -> HtHp/1
  FK Function/11(HtRHp) -> HtRHp/1
  FK Function/12(HtLHp) -> HtLHp/1
  FK Function/13(HtRK) -> HtRK/1
  FK Function/18(HtLAr) -> HtLAr/1

== system NUgus/Kinematics/Hip Roll Compensation/Inject Control Signal ==
  hrr_ref : Inport
  hrl_ref : Inport  Port=2
  theta ref1 : Inport  Port=3
  theta ref2 : Inport  Port=4
  Gain : Gain  Gain=0.6
  Gain1 : Gain  Gain=0.6
  Sum : Sum  Inputs=++|
  Sum1 : Sum  Inputs=++|
  Sum2 : Sum  Inputs=-+|
  Sum3 : Sum  Inputs=-+|
  theta p1 : Outport
  theta p2 : Outport  Port=2
  wires:
  Sum1/1 -> theta p2/1
  Gain/1 -> Sum/1
  theta ref1/1 -> Sum/2, Sum3/1
  Sum/1 -> theta p1/1
  Sum3/1 -> Gain/1
  Sum2/1 -> Gain1/1
  Gain1/1 -> Sum1/1  "theta_e"
  theta ref2/1 -> Sum1/2, Sum2/1
  hrr_ref/1 -> Sum3/2
  hrl_ref/1 -> Sum2/2

== system NUgus/Kinematics/Hip Roll Compensation/disc to rad//s ==
  disc : Inport
  Add1 : Sum  Inputs=+-
  Constant4 : Constant  Value=512
  Gain : Gain  Gain=(500*pi)/(180*512)  OutDataTypeStr=double
  rad : Outport
  wires:
  disc/1 -> Add1/1
  Gain/1 -> rad/1
  Add1/1 -> Gain/1
  Constant4/1 -> Add1/2

== system NUgus/Kinematics/Hip Roll Compensation1/Inject Control Signal ==
  hrr_ref : Inport
  hrl_ref : Inport  Port=2
  theta ref1 : Inport  Port=3
  theta ref2 : Inport  Port=4
  Gain : Gain  Gain=0.6
  Gain1 : Gain  Gain=0.6
  Sum : Sum  Inputs=++|
  Sum1 : Sum  Inputs=++|
  Sum2 : Sum  Inputs=-+|
  Sum3 : Sum  Inputs=-+|
  theta p1 : Outport
  theta p2 : Outport  Port=2
  wires:
  Sum1/1 -> theta p2/1
  Gain/1 -> Sum/1
  theta ref1/1 -> Sum/2, Sum3/1
  Sum/1 -> theta p1/1
  Sum3/1 -> Gain/1
  Sum2/1 -> Gain1/1
  Gain1/1 -> Sum1/1  "theta_e"
  theta ref2/1 -> Sum1/2, Sum2/1
  hrr_ref/1 -> Sum3/2
  hrl_ref/1 -> Sum2/2

== system NUgus/Kinematics/Hip Roll Compensation1/disc to rad//s ==
  disc : Inport
  Add1 : Sum  Inputs=+-
  Constant4 : Constant  Value=512
  Gain : Gain  Gain=(500*pi)/(180*512)  OutDataTypeStr=double
  rad : Outport
  wires:
  disc/1 -> Add1/1
  Gain/1 -> rad/1
  Add1/1 -> Gain/1
  Constant4/1 -> Add1/2

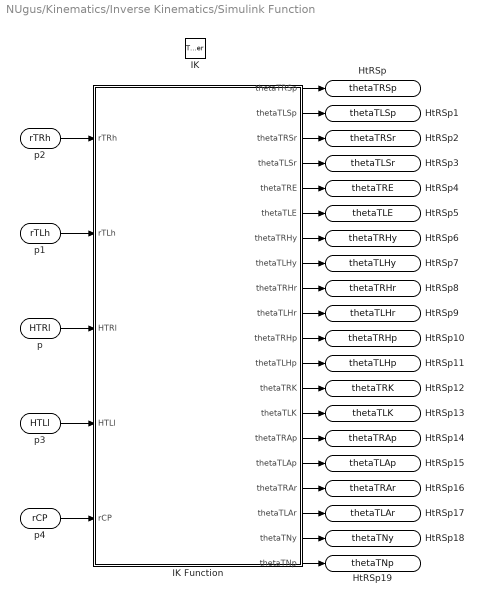
== system NUgus/Kinematics/Inverse Kinematics/Simulink Function ==
  IK : TriggerPort  TriggerType=function-call  IsSimulinkFunction=on  FunctionName=IK  FunctionVisibility=scoped  VariantControl=(inherit)
  IK Function : MATLAB Function  TreatAsAtomicUnit=on
  p2 : ArgIn  DisableCoverage=on  PortDimensions=[1 3]  ArgumentName=rTRh
  p1 : ArgIn  DisableCoverage=on  Port=2  PortDimensions=[1 3]  ArgumentName=rTLh
  p : ArgIn  DisableCoverage=on  Port=3  PortDimensions=[4 4]  ArgumentName=HTRl
  p3 : ArgIn  DisableCoverage=on  Port=4  PortDimensions=[4 4]  ArgumentName=HTLl
  p4 : ArgIn  DisableCoverage=on  Port=5  PortDimensions=[1 3]  ArgumentName=rCP
  HtRSp : ArgOut  DisableCoverage=on  ArgumentName=thetaTRSp
  HtRSp1 : ArgOut  DisableCoverage=on  Port=2  ArgumentName=thetaTLSp
  HtRSp2 : ArgOut  DisableCoverage=on  Port=3  ArgumentName=thetaTRSr
  HtRSp3 : ArgOut  DisableCoverage=on  Port=4  ArgumentName=thetaTLSr
  HtRSp4 : ArgOut  DisableCoverage=on  Port=5  ArgumentName=thetaTRE
  HtRSp5 : ArgOut  DisableCoverage=on  Port=6  ArgumentName=thetaTLE
  HtRSp6 : ArgOut  DisableCoverage=on  Port=7  ArgumentName=thetaTRHy
  HtRSp7 : ArgOut  DisableCoverage=on  Port=8  ArgumentName=thetaTLHy
  HtRSp8 : ArgOut  DisableCoverage=on  Port=9  ArgumentName=thetaTRHr
  HtRSp9 : ArgOut  DisableCoverage=on  Port=10  ArgumentName=thetaTLHr
  HtRSp10 : ArgOut  DisableCoverage=on  Port=11  ArgumentName=thetaTRHp
  HtRSp11 : ArgOut  DisableCoverage=on  Port=12  ArgumentName=thetaTLHp
  HtRSp12 : ArgOut  DisableCoverage=on  Port=13  ArgumentName=thetaTRK
  HtRSp13 : ArgOut  DisableCoverage=on  Port=14  ArgumentName=thetaTLK
  HtRSp14 : ArgOut  DisableCoverage=on  Port=15  ArgumentName=thetaTRAp
  HtRSp15 : ArgOut  DisableCoverage=on  Port=16  ArgumentName=thetaTLAp
  HtRSp16 : ArgOut  DisableCoverage=on  Port=17  ArgumentName=thetaTRAr
  HtRSp17 : ArgOut  DisableCoverage=on  Port=18  ArgumentName=thetaTLAr
  HtRSp18 : ArgOut  DisableCoverage=on  Port=19  ArgumentName=thetaTNy
  HtRSp19 : ArgOut  DisableCoverage=on  Port=20  ArgumentName=thetaTNp
  wires:
  p/1 -> IK Function/3(HTRl)
  p1/1 -> IK Function/2(rTLh)
  p2/1 -> IK Function/1(rTRh)
  p3/1 -> IK Function/4(HTLl)
  p4/1 -> IK Function/5(rCP)
  IK Function/1(thetaTRSp) -> HtRSp/1
  IK Function/2(thetaTLSp) -> HtRSp1/1
  IK Function/3(thetaTRSr) -> HtRSp2/1
  IK Function/4(thetaTLSr) -> HtRSp3/1
  IK Function/5(thetaTRE) -> HtRSp4/1
  IK Function/6(thetaTLE) -> HtRSp5/1
  IK Function/7(thetaTRHy) -> HtRSp6/1
  IK Function/8(thetaTLHy) -> HtRSp7/1
  IK Function/9(thetaTRHr) -> HtRSp8/1
  IK Function/10(thetaTLHr) -> HtRSp9/1
  IK Function/11(thetaTRHp) -> HtRSp10/1
  IK Function/12(thetaTLHp) -> HtRSp11/1
  IK Function/13(thetaTRK) -> HtRSp12/1
  IK Function/14(thetaTLK) -> HtRSp13/1
  IK Function/15(thetaTRAp) -> HtRSp14/1
  IK Function/16(thetaTLAp) -> HtRSp15/1
  IK Function/17(thetaTRAr) -> HtRSp16/1
  IK Function/18(thetaTLAr) -> HtRSp17/1
  IK Function/19(thetaTNy) -> HtRSp18/1
  IK Function/20(thetaTNp) -> HtRSp19/1

== system NUgus/Kinematics/Torso Centre of Mass/Simulink Function ==
  TorsoCOM : TriggerPort  TriggerType=function-call  IsSimulinkFunction=on  FunctionName=TorsoCOM  FunctionVisibility=scoped  VariantControl=(inherit)
  MATLAB Function : MATLAB Function  TreatAsAtomicUnit=on
  HtRSp : ArgIn  DisableCoverage=on  PortDimensions=[4 4]  ArgumentName=HtRSp
  HtLSp : ArgIn  DisableCoverage=on  Port=2  PortDimensions=[4 4]  ArgumentName=HtLSp
  HtRSr : ArgIn  DisableCoverage=on  Port=3  PortDimensions=[4 4]  ArgumentName=HtRSr
  HtLSr : ArgIn  DisableCoverage=on  Port=4  PortDimensions=[4 4]  ArgumentName=HtLSr
  HtRE : ArgIn  DisableCoverage=on  Port=5  PortDimensions=[4 4]  ArgumentName=HtRE
  HtLE : ArgIn  DisableCoverage=on  Port=6  PortDimensions=[4 4]  ArgumentName=HtLE
  HtHy : ArgIn  DisableCoverage=on  Port=7  PortDimensions=[4 4]  ArgumentName=HtHy
  HtHp : ArgIn  DisableCoverage=on  Port=8  PortDimensions=[4 4]  ArgumentName=HtHp
  com : ArgOut  DisableCoverage=on  PortDimensions=[1 3]  ArgumentName=torso_com
  mass : ArgOut  DisableCoverage=on  Port=2  ArgumentName=torso_mass
  wires:
  HtRSp/1 -> MATLAB Function/1(HtRSp)
  HtLSp/1 -> MATLAB Function/2(HtLSp)
  HtRSr/1 -> MATLAB Function/3(HtRSr)
  HtLSr/1 -> MATLAB Function/4(HtLSr)
  HtRE/1 -> MATLAB Function/5(HtRE)
  HtLE/1 -> MATLAB Function/6(HtLE)
  HtHy/1 -> MATLAB Function/7(HtHy)
  HtHp/1 -> MATLAB Function/8(HtHp)
  MATLAB Function/1(torso_com) -> com/1
  MATLAB Function/2(torso_mass) -> mass/1

== system NUgus/NUgus/6 DoF/Subsystem ==
  Mux4 : Mux  Inputs=3
  PS-Simulink Converter14 : nesl_utility/PS-Simulink Converter  PhysicalDomain=network_engine_domain  SubClassName=ps_output  LeftPortType=input  RightPortType=output  PseudoPeriodic=off  Frequencies=[]  Unit=rad/s  AffineConversion=off
  PS-Simulink Converter15 : nesl_utility/PS-Simulink Converter  PhysicalDomain=network_engine_domain  SubClassName=ps_output  LeftPortType=input  RightPortType=output  PseudoPeriodic=off  Frequencies=[]  Unit=rad/s  AffineConversion=off
  PS-Simulink Converter16 : nesl_utility/PS-Simulink Converter  PhysicalDomain=network_engine_domain  SubClassName=ps_output  LeftPortType=input  RightPortType=output  PseudoPeriodic=off  Frequencies=[]  Unit=rad/s  AffineConversion=off
  Transfer Fcn1 : TransferFcn  Numerator=[4]  Denominator=[1 4 4]
  Transfer Fcn2 : TransferFcn  Numerator=[4]  Denominator=[1 4 4]
  Transfer Fcn3 : TransferFcn  Numerator=[4]  Denominator=[1 4 4]
  wx : PMIOPort  Side=Left
  wy : PMIOPort  Port=2  Side=Left
  wz : PMIOPort  Port=3  Side=Left
  omega : Outport
  wires:
  PS-Simulink Converter14/1 -> Transfer Fcn3/1
  PS-Simulink Converter15/1 -> Transfer Fcn1/1
  Mux4/1 -> omega/1
  PS-Simulink Converter16/1 -> Transfer Fcn2/1
  Transfer Fcn2/1 -> Mux4/3
  Transfer Fcn3/1 -> Mux4/1
  Transfer Fcn1/1 -> Mux4/2
  connections:
  wy/RConn1 -- PS-Simulink Converter15/LConn1
  PS-Simulink Converter14/LConn1 -- wx/RConn1
  wz/RConn1 -- PS-Simulink Converter16/LConn1

== system NUgus/NUgus/6 DoF/Subsystem1 ==
  Mux : Mux  Inputs=3
  PS-Simulink Converter : nesl_utility/PS-Simulink Converter  PhysicalDomain=network_engine_domain  SubClassName=ps_output  LeftPortType=input  RightPortType=output  PseudoPeriodic=off  Frequencies=[]  Unit=m  AffineConversion=off
  PS-Simulink Converter6 : nesl_utility/PS-Simulink Converter  PhysicalDomain=network_engine_domain  SubClassName=ps_output  LeftPortType=input  RightPortType=output  PseudoPeriodic=off  Frequencies=[]  Unit=m  AffineConversion=off
  PS-Simulink Converter7 : nesl_utility/PS-Simulink Converter  PhysicalDomain=network_engine_domain  SubClassName=ps_output  LeftPortType=input  RightPortType=output  PseudoPeriodic=off  Frequencies=[]  Unit=m  AffineConversion=off
  px : PMIOPort  Side=Left
  py : PMIOPort  Port=2  Side=Left
  pz : PMIOPort  Port=3  Side=Left
  p : Outport
  wires:
  PS-Simulink Converter/1 -> Mux/1
  PS-Simulink Converter7/1 -> Mux/3
  Mux/1 -> p/1
  PS-Simulink Converter6/1 -> Mux/2
  connections:
  py/RConn1 -- PS-Simulink Converter6/LConn1
  px/RConn1 -- PS-Simulink Converter/LConn1
  pz/RConn1 -- PS-Simulink Converter7/LConn1

== system NUgus/NUgus/6 DoF/Subsystem2 ==
  Mux2 : Mux  Inputs=3
  PS-Simulink Converter10 : nesl_utility/PS-Simulink Converter  PhysicalDomain=network_engine_domain  SubClassName=ps_output  LeftPortType=input  RightPortType=output  PseudoPeriodic=off  Frequencies=[]  Unit=m/s  AffineConversion=off
  PS-Simulink Converter8 : nesl_utility/PS-Simulink Converter  PhysicalDomain=network_engine_domain  SubClassName=ps_output  LeftPortType=input  RightPortType=output  PseudoPeriodic=off  Frequencies=[]  Unit=m/s  AffineConversion=off
  PS-Simulink Converter9 : nesl_utility/PS-Simulink Converter  PhysicalDomain=network_engine_domain  SubClassName=ps_output  LeftPortType=input  RightPortType=output  PseudoPeriodic=off  Frequencies=[]  Unit=m/s  AffineConversion=off
  vx : PMIOPort  Side=Left
  vy : PMIOPort  Port=2  Side=Left
  vz : PMIOPort  Port=3  Side=Left
  v : Outport
  wires:
  PS-Simulink Converter8/1 -> Mux2/1
  PS-Simulink Converter10/1 -> Mux2/3
  Mux2/1 -> v/1
  PS-Simulink Converter9/1 -> Mux2/2
  connections:
  vz/RConn1 -- PS-Simulink Converter10/LConn1
  vy/RConn1 -- PS-Simulink Converter9/LConn1
  PS-Simulink Converter8/LConn1 -- vx/RConn1

== system NUgus/NUgus/6 DoF/Subsystem3 ==
  Mux3 : Mux  Inputs=3
  PS-Simulink Converter11 : nesl_utility/PS-Simulink Converter  PhysicalDomain=network_engine_domain  SubClassName=ps_output  LeftPortType=input  RightPortType=output  PseudoPeriodic=off  Frequencies=[]  Unit=m/s^2  AffineConversion=off
  PS-Simulink Converter12 : nesl_utility/PS-Simulink Converter  PhysicalDomain=network_engine_domain  SubClassName=ps_output  LeftPortType=input  RightPortType=output  PseudoPeriodic=off  Frequencies=[]  Unit=m/s^2  AffineConversion=off
  PS-Simulink Converter13 : nesl_utility/PS-Simulink Converter  PhysicalDomain=network_engine_domain  SubClassName=ps_output  LeftPortType=input  RightPortType=output  PseudoPeriodic=off  Frequencies=[]  Unit=m/s^2  AffineConversion=off
  Transfer Fcn1 : TransferFcn  Numerator=[4]  Denominator=[1 4 4]
  Transfer Fcn2 : TransferFcn  Numerator=[4]  Denominator=[1 4 4]
  Transfer Fcn3 : TransferFcn  Numerator=[4]  Denominator=[1 4 4]
  ax : PMIOPort  Side=Left
  ay : PMIOPort  Port=2  Side=Left
  az : PMIOPort  Port=3  Side=Left
  alpha : Outport
  wires:
  PS-Simulink Converter11/1 -> Transfer Fcn2/1
  PS-Simulink Converter12/1 -> Transfer Fcn3/1
  PS-Simulink Converter13/1 -> Transfer Fcn1/1
  Mux3/1 -> alpha/1
  Transfer Fcn1/1 -> Mux3/2
  Transfer Fcn2/1 -> Mux3/3
  Transfer Fcn3/1 -> Mux3/1
  connections:
  ay/RConn1 -- PS-Simulink Converter13/LConn1
  PS-Simulink Converter12/LConn1 -- ax/RConn1
  az/RConn1 -- PS-Simulink Converter11/LConn1
